simulink model "Ex6"  (R2025b)
settings: Solver=VariableStepAuto  StartTime=0.0  StopTime=10.0  RelTol=1e-3

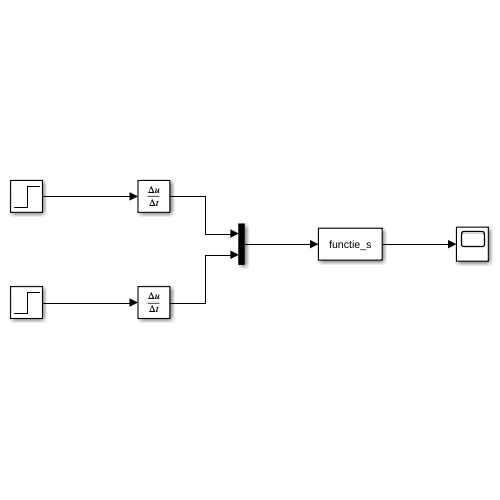
[thumbnail: Simulink's stored preview of the top-level diagram]
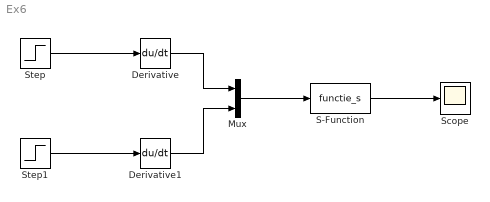
== system Ex6 ==
  Derivative : Derivative
  Derivative1 : Derivative
  Mux : Mux  Inputs=2
  S-Function : S-Function  FunctionName=functie_s  Parameters=[-1 0 0; 0 -2 1; 0 -1 -3], [1 0; 0 1; 1 -1], [1 0 1; 0 1 -1]  SFunctionDeploymentMode=off  EnableBusSupport=off
  Scope : Scope
  Step : Step  SampleTime=0
  Step1 : Step  SampleTime=0
  wires:
  Step/1 -> Derivative/1
  Step1/1 -> Derivative1/1
  Derivative/1 -> Mux/1
  Derivative1/1 -> Mux/2
  Mux/1 -> S-Function/1
  S-Function/1 -> Scope/1
